simulink model "sim5input"  (R2020a)
settings: Solver=VariableStepAuto  StartTime=0.0  StopTime=30  RelTol=1e-3
undefined symbols (not defined in the file): a, a0, a1, a10, a11, a12, a13, a14, a15, a16, a17, a2, a3, a4, a5, a6, a7, a8, a9, alpha, Area, b, b1, b11, b12, b2, bankingAngle, C_fuel, camber, curveCenters, Cx, Cz, distanceThreshold, g, init_vel, init_y_pos, IT, K_wear, l_f, l_r, m_fuel, mT, overlapThreshold, rho_0, rho_1, TyreContactArea, w1, w2
libraries: simulink x7
(part 2 of 2)

== matlab function sim5input/DynamicModel/WindEffect ==
  data: rho_0 input; aerodynamic_coeff output; rho_1 input; ego_x input; ego_y input; opp_x input; opp_y input; distanceThreshold input; overlapThreshold input; alpha input; curveCenters input
function aerodynamic_coeff = windEffect(rho_0, rho_1, ego_x, ego_y, ... 
    opp_x, opp_y, distanceThreshold, overlapThreshold, alpha, curveCenters)

%give in output rho_0 if too distant from other vehicle
%rho_1 otherwise
distanceThresholdCurve =  alpha * distanceThreshold;
overlapThresholdCurve =  alpha * overlapThreshold;

if  ego_x > curveCenters(1,1) && ego_y < curveCenters(1,2) %check if in the first curve
    ego_radius = sqrt((ego_x - curveCenters(1,1))^2 + (ego_y - curveCenters(1,2))^2);
    opp_radius = sqrt((opp_x - curveCenters(1,1))^2 + (opp_y - curveCenters(1,2))^2);
    if abs(ego_radius - opp_radius) < overlapThresholdCurve && ...
            sqrt((ego_x - opp_x)^2 + (ego_y - opp_y)^2) < distanceThresholdCurve && ...
            ego_y < opp_y
        aerodynamic_coeff = rho_1;
    else
       aerodynamic_coeff = rho_0;
    end
elseif ego_x > curveCenters(2,1) && ego_y > curveCenters(2,2) %check if in the second curve
    ego_radius = sqrt((ego_x - curveCenters(2,1))^2 + (ego_y - curveCenters(2,2))^2);
    opp_radius = sqrt((opp_x - curveCenters(2,1))^2 + (opp_y - curveCenters(2,2))^2);
    if abs(ego_radius - opp_radius) < overlapThresholdCurve && ...
            sqrt((ego_x - opp_x)^2 + (ego_y - opp_y)^2) < distanceThresholdCurve && ...
            ego_x > opp_x
        aerodynamic_coeff = rho_1;
    else
       aerodynamic_coeff = rho_0;
    end
elseif ego_x < curveCenters(3,1) && ego_y > curveCenters(3,2) %check if in the third curve
    ego_radius = sqrt((ego_x - curveCenters(3,1))^2 + (ego_y - curveCenters(3,2))^2);
    opp_radius = sqrt((opp_x - curveCenters(3,1))^2 + (opp_y - curveCenters(3,2))^2);
    if abs(ego_radius - opp_radius) < overlapThresholdCurve && ...
            sqrt((ego_x - opp_x)^2 + (ego_y - opp_y)^2) < distanceThresholdCurve && ...
            ego_y > opp_y
        aerodynamic_coeff = rho_1;
    else
       aerodynamic_coeff = rho_0;
    end
elseif ego_x < curveCenters(4,1) && ego_y < curveCenters(4,2) %check if in the fourth curve
    ego_radius = sqrt((ego_x - curveCenters(4,1))^2 + (ego_y - curveCenters(4,2))^2);
    opp_radius = sqrt((opp_x - curveCenters(4,1))^2 + (opp_y - curveCenters(4,2))^2);
    if abs(ego_radius - opp_radius) < overlapThresholdCurve && ...
            sqrt((ego_x - opp_x)^2 + (ego_y - opp_y)^2) < distanceThresholdCurve && ...
            ego_x < opp_x
        aerodynamic_coeff = rho_1;
    else
       aerodynamic_coeff = rho_0;
    end
else
    %check for which straights
    if ego_y < curveCenters(1,2) && ego_x >= curveCenters(4,1) && ego_x <= curveCenters(1,1)
       %first long straight
       if abs(ego_y - opp_y) < overlapThreshold && ...
               abs(opp_x - ego_x) < distanceThreshold && ...
               ego_x < opp_x
           aerodynamic_coeff = rho_1;
       else
           aerodynamic_coeff = rho_0;
       end
       
    elseif ego_y > curveCenters(2,2) && ego_x >= curveCenters(3,1) && ego_x <= curveCenters(2,1)
       %second long straight
       if abs(ego_y - opp_y) < overlapThreshold && ...
               abs(opp_x - ego_x) < distanceThreshold && ...
               ego_x > opp_x
           aerodynamic_coeff = rho_1;
       else
           aerodynamic_coeff = rho_0;
       end
       
    elseif ego_x > curveCenters(1,1) && ego_y >= curveCenters(1,2) && ego_y <= curveCenters(2,2)
       %first short straight
       if abs(ego_x - opp_x) < overlapThreshold && ...
               abs(opp_y - ego_y) < distanceThreshold && ...
               ego_y < opp_y
           aerodynamic_coeff = rho_1;
       else
           aerodynamic_coeff = rho_0;
       end
       
    elseif ego_x < curveCenters(3,1) && ego_y >= curveCenters(4,2) && ego_y <= curveCenters(3,2)
       %second short straight
       if abs(ego_x - opp_x) < overlapThreshold && ...
               abs(opp_y - ego_y) < distanceThreshold && ...
               ego_y > opp_y
           aerodynamic_coeff = rho_1;
       else
           aerodynamic_coeff = rho_0;
       end
       
    else
        aerodynamic_coeff = rho_0;
    end
end
